simulink model "PID_1"  (R2023b)
settings: Solver=VariableStepAuto  StartTime=0.0  StopTime=10.0  RelTol=1e-3
undefined symbols (not defined in the file): KI, KP
settings Model: Creator=yeoseojeong  LastModifiedBy=yeoseojeong

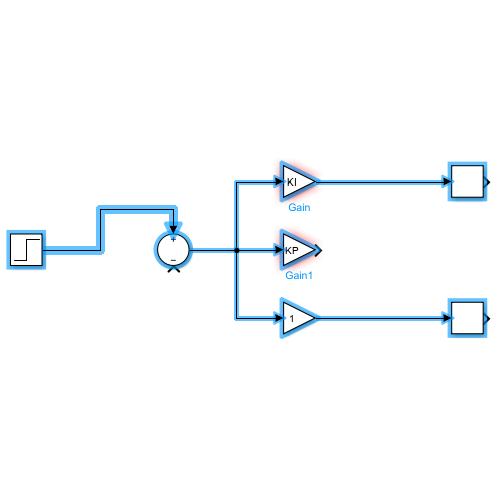
[thumbnail: Simulink's stored preview of the top-level diagram]
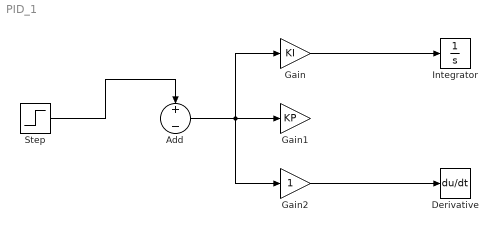
== system PID_1 ==
  Add : Sum  Inputs=+-
  Derivative : Derivative
  Gain : Gain  Gain=KI
  Gain1 : Gain  Gain=KP
  Gain2 : Gain
  Integrator : Integrator
  Step : Step  SampleTime=0
  wires:
  Gain/1 -> Integrator/1
  Add/1 -> Gain1/1, Gain2/1, Gain/1
  Gain2/1 -> Derivative/1
  Step/1 -> Add/1
